simulink model "Droop_Ctrl"  (R2022b)
settings: Solver=ode113  StartTime=0.0  StopTime=1.5  RelTol=1e-3  EnableMultiTasking=on
libraries: spsSeriesRLCBranchLib x12, powerlib_extras x11, spsThreePhaseVIMeasurementLib x8, spsThreePhaseBreakerLib x7, spsThreePhaseSeriesRLCLoadLib x4, spsabctodq0Lib x4, spsDCVoltageSourceLib x2, spsThreePhaseSeriesRLCBranchLib x2, spsUniversalBridgeLib x2, spsdq0toabcLib x1, spspowerguiLib x1
settings Model: SimulationMode=accelerator  Creator=Administrator  LastModifiedBy=Rov
settings SolverCC: AlgebraicLoopSolver=TrustRegion
settings DataIOCC: LimitDataPoints=on  SaveFormat=Array  ReturnWorkspaceOutputs=off
settings OptimizationCC: ExpressionDepthLimit=2147483647  LifeSpan=inf
settings DebuggingCC: UnderspecifiedInitializationDetection=Classic  MergeDetectMultiDrivingBlocksExec=none  SolverPrmCheckMsg=warning  UnconnectedInputMsg=warning  UnconnectedOutputMsg=warning  UnconnectedLineMsg=warning  AllowSymbolicDim=off  StateNameClashWarn=warning  SFUnexpectedBacktrackingDiag=warning  SFNoUnconditionalDefaultTransitionDiag=warning  SFExecutionAtInitializationDiag=none  SFMachineParentedDataDiag=warning  ArithmeticOperatorsInVariantConditions=warning
settings HardwareCC: ProdBitPerPointer=32  ProdBitPerSizeT=32  ProdBitPerPtrDiffT=32  ProdLargestAtomicFloat=None  ProdIntDivRoundTo=Undefined  ProdEndianess=Unspecified  ProdWordSize=32  ProdHWDeviceType=32-bit Generic
settings ModelReferenceCC: EnableRefExpFcnMdlSchedulingChecks=on  PropagateSignalLabelsOutOfModel=off
settings SFSimCC: SimUseLocalCustomCode=off  CustomCodeUndefinedFunction=UseInterfaceOnly
settings RTWCC: RTWUseLocalCustomCode=off
settings CodeAppCC: StateflowObjectComments=on
settings GRTTargetCC: TargetLangStandard=C89/C90 (ANSI)
settings ConfigComp: CovMetricSettings=dw  CovSaveCumulativeToWorkspaceVar=on  CovSaveSingleToWorkspaceVar=on  CovExternalEMLEnable=off
settings SimscapeCC: SimscapeNormalizeSystem=off

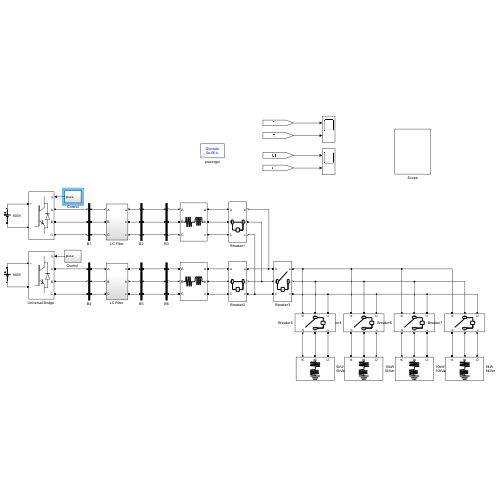
[thumbnail: Simulink's stored preview of the top-level diagram]
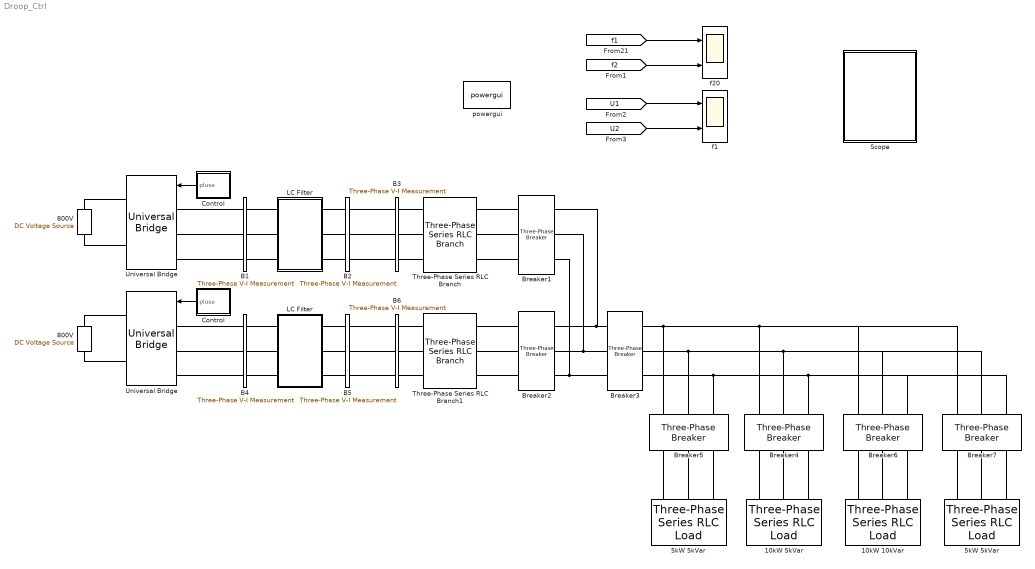
== system Droop_Ctrl ==
  10kW 10kVar : spsThreePhaseSeriesRLCLoadLib/Three-Phase Series RLC Load  LConnTagsString=A|B|C  Configuration=Y (grounded)  NominalVoltage=380  Vabc=[1e3 1e3 1e3]  Vabcp=[1e3 1e3 1e3]  NominalFrequency=50  UnbalancedPower=off  ActivePower=10e3  InductivePower=10e3  CapacitivePower=0  Pabc=[10e3 9e3 11e3]  QLabc=[100 90 110]  QCabc=[100 90 110]  Pabcp=[10e3 9e3 11e3]  QLabcp=[100 90 110]  QCabcp=[100 90 110]  Measurements=None  LoadType=constant Z
  10kW 5kVar : spsThreePhaseSeriesRLCLoadLib/Three-Phase Series RLC Load  LConnTagsString=A|B|C  Configuration=Y (grounded)  NominalVoltage=380  Vabc=[1e3 1e3 1e3]  Vabcp=[1e3 1e3 1e3]  NominalFrequency=50  UnbalancedPower=off  ActivePower=10e3  InductivePower=5e3  CapacitivePower=0  Pabc=[10e3 9e3 11e3]  QLabc=[100 90 110]  QCabc=[100 90 110]  Pabcp=[10e3 9e3 11e3]  QLabcp=[100 90 110]  QCabcp=[100 90 110]  Measurements=None  LoadType=constant Z
  5kW 5kVar : spsThreePhaseSeriesRLCLoadLib/Three-Phase Series RLC Load  LConnTagsString=A|B|C  Configuration=Y (grounded)  NominalVoltage=380  Vabc=[1e3 1e3 1e3]  Vabcp=[1e3 1e3 1e3]  NominalFrequency=50  UnbalancedPower=off  ActivePower=5e3  InductivePower=5e3  CapacitivePower=0  Pabc=[10e3 9e3 11e3]  QLabc=[100 90 110]  QCabc=[100 90 110]  Pabcp=[10e3 9e3 11e3]  QLabcp=[100 90 110]  QCabcp=[100 90 110]  Measurements=None  LoadType=constant Z
  "5kW 5kVar " : spsThreePhaseSeriesRLCLoadLib/Three-Phase Series RLC Load  LConnTagsString=A|B|C  Configuration=Y (grounded)  NominalVoltage=380  Vabc=[1e3 1e3 1e3]  Vabcp=[1e3 1e3 1e3]  NominalFrequency=50  UnbalancedPower=off  ActivePower=5e3  InductivePower=5e3  CapacitivePower=0  Pabc=[10e3 9e3 11e3]  QLabc=[100 90 110]  QCabc=[100 90 110]  Pabcp=[10e3 9e3 11e3]  QLabcp=[100 90 110]  QCabcp=[100 90 110]  Measurements=None  LoadType=constant Z
  800V : spsDCVoltageSourceLib/DC Voltage Source  Amplitude=800  Measurements=None
  "800V " : spsDCVoltageSourceLib/DC Voltage Source  Amplitude=800  Measurements=None
  B1 : spsThreePhaseVIMeasurementLib/Three-Phase V-I Measurement  VoltageMeasurement=phase-to-ground  SetLabelV=on  LabelV=Vabc_B1  Vpu=off  VpuLL=off  CurrentMeasurement=yes  SetLabelI=on  LabelI=Iabc_B1  Ipu=off  Pbase=100e6  Vbase=500e3  OutputType=Complex  PhasorSimulation=off  PSBequivalent=0
  B2 : spsThreePhaseVIMeasurementLib/Three-Phase V-I Measurement  VoltageMeasurement=phase-to-ground  SetLabelV=on  LabelV=Vabc_B2  Vpu=off  VpuLL=off  CurrentMeasurement=yes  SetLabelI=on  LabelI=Iabc_B2  Ipu=off  Pbase=100e6  Vbase=500e3  OutputType=Complex  PhasorSimulation=off  PSBequivalent=0
  B3 : spsThreePhaseVIMeasurementLib/Three-Phase V-I Measurement  VoltageMeasurement=phase-to-ground  SetLabelV=on  LabelV=Vabc_B3  Vpu=off  VpuLL=off  CurrentMeasurement=yes  SetLabelI=on  LabelI=Iabc_B3  Ipu=off  Pbase=100e6  Vbase=500e3  OutputType=Complex  PhasorSimulation=off  PSBequivalent=0
  B4 : spsThreePhaseVIMeasurementLib/Three-Phase V-I Measurement  VoltageMeasurement=phase-to-ground  SetLabelV=on  LabelV=Vabc_B4  Vpu=off  VpuLL=off  CurrentMeasurement=yes  SetLabelI=on  LabelI=Iabc_B4  Ipu=off  Pbase=100e6  Vbase=500e3  OutputType=Complex  PhasorSimulation=off  PSBequivalent=0
  B5 : spsThreePhaseVIMeasurementLib/Three-Phase V-I Measurement  VoltageMeasurement=phase-to-ground  SetLabelV=on  LabelV=Vabc_B5  Vpu=off  VpuLL=off  CurrentMeasurement=yes  SetLabelI=on  LabelI=Iabc_B5  Ipu=off  Pbase=100e6  Vbase=500e3  OutputType=Complex  PhasorSimulation=off  PSBequivalent=0
  B6 : spsThreePhaseVIMeasurementLib/Three-Phase V-I Measurement  VoltageMeasurement=phase-to-ground  SetLabelV=on  LabelV=Vabc_B6  Vpu=off  VpuLL=off  CurrentMeasurement=yes  SetLabelI=on  LabelI=Iabc_B6  Ipu=off  Pbase=100e6  Vbase=500e3  OutputType=Complex  PhasorSimulation=off  PSBequivalent=0
  Breaker1 : spsThreePhaseBreakerLib/Three-Phase Breaker  InitialState=closed  SwitchA=on  SwitchB=on  SwitchC=on  SwitchTimes=[10 10.4]  External=off  BreakerResistance=0.001  SnubberResistance=1e6  SnubberCapacitance=inf  Measurements=None
  Breaker2 : spsThreePhaseBreakerLib/Three-Phase Breaker  InitialState=closed  SwitchA=on  SwitchB=on  SwitchC=on  SwitchTimes=[10 10.4]  External=off  BreakerResistance=0.001  SnubberResistance=1e6  SnubberCapacitance=inf  Measurements=None
  Breaker3 : spsThreePhaseBreakerLib/Three-Phase Breaker  InitialState=open  SwitchA=on  SwitchB=on  SwitchC=on  SwitchTimes=[0.2 10]  External=off  BreakerResistance=0.001  SnubberResistance=1e6  SnubberCapacitance=inf  Measurements=None
  Breaker4 : spsThreePhaseBreakerLib/Three-Phase Breaker  InitialState=open  SwitchA=on  SwitchB=on  SwitchC=on  SwitchTimes=[0.4 0.6]  External=off  BreakerResistance=0.001  SnubberResistance=1e6  SnubberCapacitance=inf  Measurements=None
  Breaker5 : spsThreePhaseBreakerLib/Three-Phase Breaker  InitialState=open  SwitchA=on  SwitchB=on  SwitchC=on  SwitchTimes=[0.2 0.4]  External=off  BreakerResistance=0.001  SnubberResistance=1e6  SnubberCapacitance=inf  Measurements=None
  Breaker6 : spsThreePhaseBreakerLib/Three-Phase Breaker  InitialState=open  SwitchA=on  SwitchB=on  SwitchC=on  SwitchTimes=[0.6 0.8]  External=off  BreakerResistance=0.001  SnubberResistance=1e6  SnubberCapacitance=inf  Measurements=None
  Breaker7 : spsThreePhaseBreakerLib/Three-Phase Breaker  InitialState=open  SwitchA=on  SwitchB=on  SwitchC=on  SwitchTimes=[0.8 1]  External=off  BreakerResistance=0.001  SnubberResistance=1e6  SnubberCapacitance=inf  Measurements=None
  Control : Subsystem
  "Control " : Subsystem
  LC Filter : Subsystem
  "LC Filter " : Subsystem
  Scope : Subsystem
  Three-Phase Series RLC Branch : spsThreePhaseSeriesRLCBranchLib/Three-Phase Series RLC Branch  LConnTagsString=A|B|C  RConnTagsString=A|B|C  BranchType=RL  Resistance=0.642/5  Inductance=0.37e-3  Capacitance=1e-6  Measurements=None
  Three-Phase Series RLC Branch1 : spsThreePhaseSeriesRLCBranchLib/Three-Phase Series RLC Branch  LConnTagsString=A|B|C  RConnTagsString=A|B|C  BranchType=RL  Resistance=0.642/5  Inductance=0.37e-3  Capacitance=1e-6  Measurements=None
  Universal Bridge : spsUniversalBridgeLib/Universal Bridge  Arms=3  SnubberResistance=1e5  SnubberCapacitance=inf  Device=IGBT / Diodes  Ron=1e-3  Lon=0  ForwardVoltages="[  0  0  ]"  ForwardVoltage=0  GTOparameters=[ 10e-6 , 20e-6 ]  IGBTparameters=[ 1e-6 , 2e-6 ]  Measurements=None  Measurements_2=None  converterType=Rectifier
  "Universal Bridge " : spsUniversalBridgeLib/Universal Bridge  Arms=3  SnubberResistance=1e5  SnubberCapacitance=inf  Device=IGBT / Diodes  Ron=1e-3  Lon=0  ForwardVoltages="[  0  0  ]"  ForwardVoltage=0  GTOparameters=[ 10e-6 , 20e-6 ]  IGBTparameters=[ 1e-6 , 2e-6 ]  Measurements=None  Measurements_2=None  converterType=Rectifier
  f1 : Scope  NumInputPorts=2
  f20 : Scope  NumInputPorts=2
  powergui : spspowerguiLib/powergui  Priority=1  SimulationMode=Discrete  SampleTime=5e-6  frequency=60  Iterations=50  frequencyindice=0  Pbase=100e6  ErrMax=1e-4  UnitsV=kV  UnitsW=MW  buscounter=0  FunctionMessages=off  echomessages=off  EnableUseOfTLC=off  CurrentSourceSwitches=off  DisableSnubberDevices=off  DisableRonSwitches=off  DisableVfSwitches=off  DisplayEquations=off  AutomaticDiscreteSolvers=off  SolverType=Tustin  Interpol=off  ExternalGateDelay=off  methode=off  Ts=100  x0status=blocks  SPID=off  SwTol=0  HookPort=off  NonlinearTolerance=1e-4  nMaxIteration=100  ContinueOnMaxIteration=off  RestoreLinks=warning  ResistiveCurrentMeasurement=off  Frange=[0:2:500]  Ylog=off  Xlog=on  ShowGrid=off  save=off  variable=ZData  structure=0  ZoomFFT=off  StartTime=0.0  cycles=1  DisplayStyle=1  fundamental=60  FreqAxis=off  MaxFrequency=1000  frequencyindicesteady=1  RmsSteady=1  display=off
  wires:
  Control/1(pluse) -> Universal Bridge/1
  "Control "/1(pluse) -> "Universal Bridge "/1
  [f1] -> f20/1
  [f2] -> f20/2
  [U1] -> f1/1
  [U2] -> f1/2
  connections:
  B2/RConn3 -- B3/LConn3
  B2/RConn2 -- B3/LConn2
  B2/RConn1 -- B3/LConn1
  800V/LConn1 -- Universal Bridge/RConn2
  800V/RConn1 -- Universal Bridge/RConn1
  Universal Bridge/LConn1 -- B1/LConn1
  Universal Bridge/LConn2 -- B1/LConn2
  Universal Bridge/LConn3 -- B1/LConn3
  Three-Phase Series RLC Branch/LConn3 -- B3/RConn3
  Three-Phase Series RLC Branch/LConn2 -- B3/RConn2
  Three-Phase Series RLC Branch/LConn1 -- B3/RConn1
  B1/RConn1 -- LC Filter/LConn1
  B2/LConn1 -- LC Filter/RConn1
  B1/RConn2 -- LC Filter/LConn2
  B2/LConn2 -- LC Filter/RConn2
  B1/RConn3 -- LC Filter/LConn3
  B2/LConn3 -- LC Filter/RConn3
  B5/RConn3 -- B6/LConn3
  B5/RConn2 -- B6/LConn2
  B5/RConn1 -- B6/LConn1
  B5/LConn3 -- "LC Filter "/RConn3
  Three-Phase Series RLC Branch1/LConn1 -- B6/RConn1
  Three-Phase Series RLC Branch1/LConn3 -- B6/RConn3
  "Universal Bridge "/LConn1 -- B4/LConn1
  "Universal Bridge "/LConn3 -- B4/LConn3
  B4/RConn1 -- "LC Filter "/LConn1
  "800V "/LConn1 -- "Universal Bridge "/RConn2
  B5/LConn2 -- "LC Filter "/RConn2
  "Universal Bridge "/LConn2 -- B4/LConn2
  Three-Phase Series RLC Branch1/LConn2 -- B6/RConn2
  "800V "/RConn1 -- "Universal Bridge "/RConn1
  B5/LConn1 -- "LC Filter "/RConn1
  B4/RConn2 -- "LC Filter "/LConn2
  B4/RConn3 -- "LC Filter "/LConn3
  Breaker2/RConn1 -- Breaker1/RConn1 -- Breaker3/LConn1
  Breaker1/RConn2 -- Breaker3/LConn2 -- Breaker2/RConn2
  Breaker1/RConn3 -- Breaker3/LConn3 -- Breaker2/RConn3
  Breaker1/LConn1 -- Three-Phase Series RLC Branch/RConn1
  Breaker1/LConn2 -- Three-Phase Series RLC Branch/RConn2
  Breaker1/LConn3 -- Three-Phase Series RLC Branch/RConn3
  Breaker2/LConn1 -- Three-Phase Series RLC Branch1/RConn1
  Breaker2/LConn2 -- Three-Phase Series RLC Branch1/RConn2
  Breaker2/LConn3 -- Three-Phase Series RLC Branch1/RConn3
  10kW 5kVar/LConn1 -- Breaker4/RConn1
  10kW 5kVar/LConn2 -- Breaker4/RConn2
  10kW 5kVar/LConn3 -- Breaker4/RConn3
  5kW 5kVar/LConn2 -- Breaker5/RConn2
  5kW 5kVar/LConn3 -- Breaker5/RConn3
  5kW 5kVar/LConn1 -- Breaker5/RConn1
  Breaker3/RConn1 -- Breaker7/LConn1 -- Breaker6/LConn1 -- Breaker4/LConn1 -- Breaker5/LConn1
  Breaker3/RConn2 -- Breaker7/LConn2 -- Breaker6/LConn2 -- Breaker4/LConn2 -- Breaker5/LConn2
  Breaker3/RConn3 -- Breaker5/LConn3 -- Breaker4/LConn3 -- Breaker6/LConn3 -- Breaker7/LConn3
  10kW 10kVar/LConn3 -- Breaker6/RConn3
  10kW 10kVar/LConn2 -- Breaker6/RConn2
  10kW 10kVar/LConn1 -- Breaker6/RConn1
  "5kW 5kVar "/LConn1 -- Breaker7/RConn1
  "5kW 5kVar "/LConn2 -- Breaker7/RConn2
  "5kW 5kVar "/LConn3 -- Breaker7/RConn3

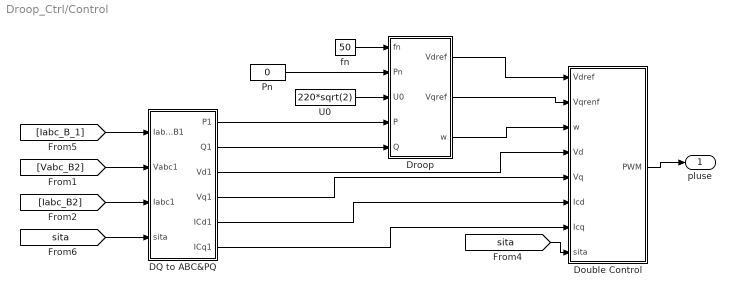
== system Droop_Ctrl/Control ==
  DQ to ABC&PQ : Subsystem
  Double Control : Subsystem
  Droop : Subsystem
  Pn : Constant  Value=0
  U0 : Constant  Value=220*sqrt(2)
  fn : Constant  Value=50
  pluse : Outport  VectorParamsAs1DForOutWhenUnconnected=off
  wires:
  Droop/3(w) -> Double Control/3(w)
  Double Control/1(PWM) -> pluse/1
  Droop/2(Vqref) -> Double Control/2(Vqrenf)
  Droop/1(Vdref) -> Double Control/1(Vdref)
  Pn/1 -> Droop/2(Pn)
  U0/1 -> Droop/3(U0)
  fn/1 -> Droop/1(fn)
  [sita] -> Double Control/8(sita)
  [sita] -> DQ to ABC&PQ/4(sita)
  [Vabc_B2] -> DQ to ABC&PQ/2(Vabc1)
  [Iabc_B2] -> DQ to ABC&PQ/3(Iabc1)
  [Iabc_B_1] -> DQ to ABC&PQ/1(Iabc_B1)
  DQ to ABC&PQ/6(ICq1) -> Double Control/7(Icq)
  DQ to ABC&PQ/5(ICd1) -> Double Control/6(Icd)
  DQ to ABC&PQ/4(Vq1) -> Double Control/5(Vq)
  DQ to ABC&PQ/3(Vd1) -> Double Control/4(Vd)
  DQ to ABC&PQ/2(Q1) -> Droop/5(Q)
  DQ to ABC&PQ/1(P1) -> Droop/4(P)

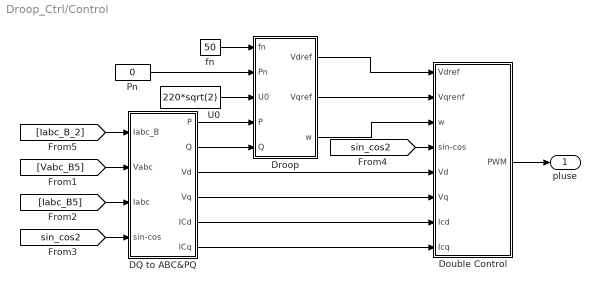
== system Droop_Ctrl/Control  ==
  DQ to ABC&PQ : Subsystem
  Double Control : Subsystem
  Droop : Subsystem
  Pn : Constant  Value=0
  U0 : Constant  Value=220*sqrt(2)
  fn : Constant  Value=50
  pluse : Outport  VectorParamsAs1DForOutWhenUnconnected=off
  wires:
  DQ to ABC&PQ/5(ICd) -> Double Control/7(Icd)
  Droop/3(w) -> Double Control/3(w)
  Double Control/1(PWM) -> pluse/1
  Droop/2(Vqref) -> Double Control/2(Vqrenf)
  Droop/1(Vdref) -> Double Control/1(Vdref)
  DQ to ABC&PQ/3(Vd) -> Double Control/5(Vd)
  DQ to ABC&PQ/6(ICq) -> Double Control/8(Icq)
  Pn/1 -> Droop/2(Pn)
  U0/1 -> Droop/3(U0)
  [Vabc_B5] -> DQ to ABC&PQ/2(Vabc)
  DQ to ABC&PQ/4(Vq) -> Double Control/6(Vq)
  DQ to ABC&PQ/1(P) -> Droop/4(P)
  [Iabc_B_2] -> DQ to ABC&PQ/1(Iabc_B)
  fn/1 -> Droop/1(fn)
  DQ to ABC&PQ/2(Q) -> Droop/5(Q)
  [Iabc_B5] -> DQ to ABC&PQ/3(Iabc)
  [sin_cos2] -> DQ to ABC&PQ/4(sin-cos)
  [sin_cos2] -> Double Control/4(sin-cos)

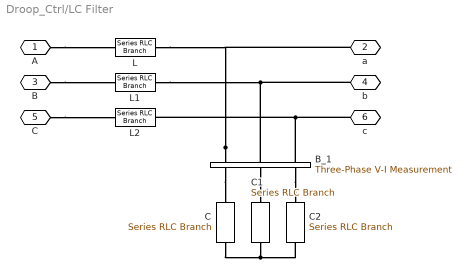
== system Droop_Ctrl/LC Filter ==
  " B_1" : spsThreePhaseVIMeasurementLib/Three-Phase V-I Measurement  VoltageMeasurement=phase-to-ground  SetLabelV=on  LabelV=Vabc_B_1  Vpu=off  VpuLL=off  CurrentMeasurement=yes  SetLabelI=on  LabelI=Iabc_B_1  Ipu=off  Pbase=100e6  Vbase=500e3  OutputType=Complex  PhasorSimulation=off  PSBequivalent=0
  C : spsSeriesRLCBranchLib/Series RLC Branch  LConnTagsString=__new0  RConnTagsString=__new0  BranchType=C  Resistance=0.01  Inductance=1e-3  SetiL0=off  InitialCurrent=0  Capacitance=1500e-6  Setx0=off  InitialVoltage=0  Measurements=None
  C1 : spsSeriesRLCBranchLib/Series RLC Branch  LConnTagsString=__new0  RConnTagsString=__new0  BranchType=C  Resistance=0.01  Inductance=1e-3  SetiL0=off  InitialCurrent=0  Capacitance=1500e-6  Setx0=off  InitialVoltage=0  Measurements=None
  C2 : spsSeriesRLCBranchLib/Series RLC Branch  LConnTagsString=__new0  RConnTagsString=__new0  BranchType=C  Resistance=0.01  Inductance=1e-3  SetiL0=off  InitialCurrent=0  Capacitance=1500e-6  Setx0=off  InitialVoltage=0  Measurements=None
  L : spsSeriesRLCBranchLib/Series RLC Branch  LConnTagsString=__new0  RConnTagsString=__new0  BranchType=L  Resistance=0.01  Inductance=2e-3  SetiL0=off  InitialCurrent=0  Capacitance=1e-6  Setx0=off  InitialVoltage=0  Measurements=None
  L1 : spsSeriesRLCBranchLib/Series RLC Branch  LConnTagsString=__new0  RConnTagsString=__new0  BranchType=L  Resistance=0.01  Inductance=2e-3  SetiL0=off  InitialCurrent=0  Capacitance=1e-6  Setx0=off  InitialVoltage=0  Measurements=None
  L2 : spsSeriesRLCBranchLib/Series RLC Branch  LConnTagsString=__new0  RConnTagsString=__new0  BranchType=L  Resistance=0.01  Inductance=2e-3  SetiL0=off  InitialCurrent=0  Capacitance=1e-6  Setx0=off  InitialVoltage=0  Measurements=None
  A : PMIOPort  Side=Left
  a : PMIOPort  Port=2  Side=Right
  B : PMIOPort  Port=3  Side=Left
  b : PMIOPort  Port=4  Side=Right
  "C " : PMIOPort  Port=5  Side=Left
  c : PMIOPort  Port=6  Side=Right
  connections:
  " B_1"/LConn1 -- a/RConn1 -- L/RConn1
  " B_1"/LConn3 -- c/RConn1 -- L2/RConn1
  A/RConn1 -- L/LConn1
  " B_1"/RConn2 -- C1/LConn1
  " B_1"/RConn3 -- C2/LConn1
  C1/RConn1 -- C/RConn1 -- C2/RConn1
  "C "/RConn1 -- L2/LConn1
  B/RConn1 -- L1/LConn1
  " B_1"/LConn2 -- b/RConn1 -- L1/RConn1
  " B_1"/RConn1 -- C/LConn1

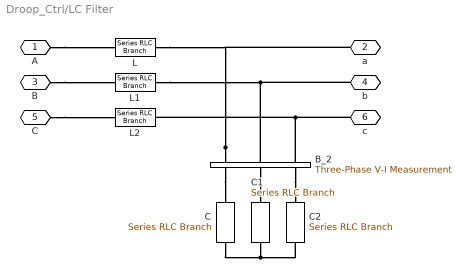
== system Droop_Ctrl/LC Filter  ==
  " B_2" : spsThreePhaseVIMeasurementLib/Three-Phase V-I Measurement  VoltageMeasurement=phase-to-ground  SetLabelV=on  LabelV=Vabc_B_2  Vpu=off  VpuLL=off  CurrentMeasurement=yes  SetLabelI=on  LabelI=Iabc_B_2  Ipu=off  Pbase=100e6  Vbase=500e3  OutputType=Complex  PhasorSimulation=off  PSBequivalent=0
  C : spsSeriesRLCBranchLib/Series RLC Branch  LConnTagsString=__new0  RConnTagsString=__new0  BranchType=C  Resistance=0.01  Inductance=1e-3  SetiL0=off  InitialCurrent=0  Capacitance=1500e-6  Setx0=off  InitialVoltage=0  Measurements=None
  C1 : spsSeriesRLCBranchLib/Series RLC Branch  LConnTagsString=__new0  RConnTagsString=__new0  BranchType=C  Resistance=0.01  Inductance=1e-3  SetiL0=off  InitialCurrent=0  Capacitance=1500e-6  Setx0=off  InitialVoltage=0  Measurements=None
  C2 : spsSeriesRLCBranchLib/Series RLC Branch  LConnTagsString=__new0  RConnTagsString=__new0  BranchType=C  Resistance=0.01  Inductance=1e-3  SetiL0=off  InitialCurrent=0  Capacitance=1500e-6  Setx0=off  InitialVoltage=0  Measurements=None
  L : spsSeriesRLCBranchLib/Series RLC Branch  LConnTagsString=__new0  RConnTagsString=__new0  BranchType=L  Resistance=0.01  Inductance=2e-3  SetiL0=off  InitialCurrent=0  Capacitance=1e-6  Setx0=off  InitialVoltage=0  Measurements=None
  L1 : spsSeriesRLCBranchLib/Series RLC Branch  LConnTagsString=__new0  RConnTagsString=__new0  BranchType=L  Resistance=0.01  Inductance=2e-3  SetiL0=off  InitialCurrent=0  Capacitance=1e-6  Setx0=off  InitialVoltage=0  Measurements=None
  L2 : spsSeriesRLCBranchLib/Series RLC Branch  LConnTagsString=__new0  RConnTagsString=__new0  BranchType=L  Resistance=0.01  Inductance=2e-3  SetiL0=off  InitialCurrent=0  Capacitance=1e-6  Setx0=off  InitialVoltage=0  Measurements=None
  A : PMIOPort  Side=Left
  a : PMIOPort  Port=2  Side=Right
  B : PMIOPort  Port=3  Side=Left
  b : PMIOPort  Port=4  Side=Right
  "C " : PMIOPort  Port=5  Side=Left
  c : PMIOPort  Port=6  Side=Right
  connections:
  " B_2"/LConn1 -- a/RConn1 -- L/RConn1
  " B_2"/LConn3 -- c/RConn1 -- L2/RConn1
  A/RConn1 -- L/LConn1
  " B_2"/RConn2 -- C1/LConn1
  " B_2"/RConn3 -- C2/LConn1
  C1/RConn1 -- C/RConn1 -- C2/RConn1
  "C "/RConn1 -- L2/LConn1
  B/RConn1 -- L1/LConn1
  " B_2"/LConn2 -- b/RConn1 -- L1/RConn1
  " B_2"/RConn1 -- C/LConn1

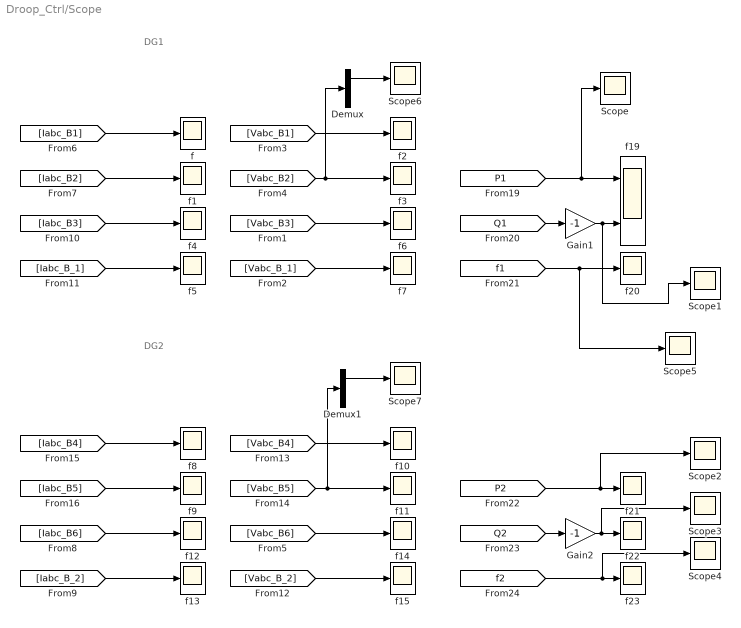
== system Droop_Ctrl/Scope ==
  note: DG1
  note: DG2
  Demux : Demux  Outputs=3
  Demux1 : Demux  Outputs=3
  Gain1 : Gain  Gain=-1
  Gain2 : Gain  Gain=-1
  Scope{,1..7} (8 alike) : Scope
  f{,1..15,20..23} (20 alike) : Scope
  f19 : Scope  NumInputPorts=2
  wires:
  [Vabc_B1] -> f2/1
  [Iabc_B3] -> f4/1
  [Vabc_B2] -> f3/1, Demux/1
  [Iabc_B1] -> f/1
  [Iabc_B2] -> f1/1
  [Iabc_B_1] -> f5/1
  [Vabc_B3] -> f6/1
  [Vabc_B_1] -> f7/1
  [Iabc_B4] -> f8/1
  [Vabc_B4] -> f10/1
  [Vabc_B6] -> f14/1
  [Iabc_B6] -> f12/1
  [Iabc_B5] -> f9/1
  [Iabc_B_2] -> f13/1
  [Vabc_B_2] -> f15/1
  [Q1] -> Gain1/1
  [P1] -> Scope/1, f19/1
  Gain1/1 -> Scope1/1, f19/2
  [f1] -> Scope5/1, f20/1
  [Q2] -> Gain2/1
  [P2] -> Scope2/1, f21/1
  Gain2/1 -> Scope3/1, f22/1
  [f2] -> Scope4/1, f23/1
  Demux/1 -> Scope6/1
  Demux1/1 -> Scope7/1
  [Vabc_B5] -> f11/1, Demux1/1

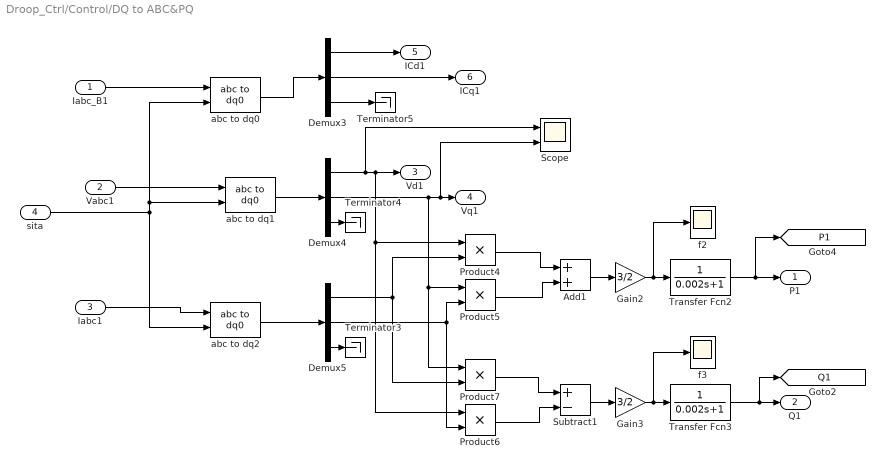
== system Droop_Ctrl/Control/DQ to ABC&PQ ==
  Iabc_B1 : Inport
  Vabc1 : Inport  Port=2
  Iabc1 : Inport  Port=3
  sita : Inport  Port=4
  Add1 : Sum
  Demux3 : Demux  Outputs=3
  Demux4 : Demux  Outputs=3
  Demux5 : Demux  Outputs=3
  Gain2 : Gain  Gain=3/2
  Gain3 : Gain  Gain=3/2
  Product{4..7} (4 alike) : Product  RndMeth=Zero
  Scope : Scope  NumInputPorts=2
  Subtract1 : Sum  Inputs=+-
  Terminator3 : Terminator
  Terminator4 : Terminator
  Terminator5 : Terminator
  Transfer Fcn2 : TransferFcn  Denominator=[0.002 1]
  Transfer Fcn3 : TransferFcn  Denominator=[0.002 1]
  abc to dq0 : spsabctodq0Lib/abc to dq0  Alignment=90 degrees behind phase A axis
  abc to dq1 : spsabctodq0Lib/abc to dq0  Alignment=90 degrees behind phase A axis
  abc to dq2 : spsabctodq0Lib/abc to dq0  Alignment=90 degrees behind phase A axis
  f2 : Scope
  f3 : Scope
  P1 : Outport  VectorParamsAs1DForOutWhenUnconnected=off
  Q1 : Outport  Port=2  VectorParamsAs1DForOutWhenUnconnected=off
  Vd1 : Outport  Port=3  VectorParamsAs1DForOutWhenUnconnected=off
  Vq1 : Outport  Port=4  VectorParamsAs1DForOutWhenUnconnected=off
  ICd1 : Outport  Port=5  VectorParamsAs1DForOutWhenUnconnected=off
  ICq1 : Outport  Port=6  VectorParamsAs1DForOutWhenUnconnected=off
  tag scope: P1=global, Q1=global
  wires:
  Demux3/3 -> Terminator5/1
  Demux5/1 -> Product7/2, Product4/2
  Add1/1 -> Gain2/1
  Gain3/1 -> f3/1, Transfer Fcn3/1
  Demux3/2 -> ICq1/1
  Product4/1 -> Add1/1
  Demux4/2 -> Scope/2, Vq1/1, Product7/1, Product5/1
  Vabc1/1 -> abc to dq1/1
  Product5/1 -> Add1/2
  abc to dq2/1 -> Demux5/1
  Demux4/1 -> Scope/1, Vd1/1, Product6/1, Product4/1
  Demux5/3 -> Terminator3/1
  Demux3/1 -> ICd1/1
  Demux4/3 -> Terminator4/1
  Gain2/1 -> f2/1, Transfer Fcn2/1
  Iabc_B1/1 -> abc to dq0/1
  Transfer Fcn2/1 -> [P1], P1/1
  Transfer Fcn3/1 -> [Q1], Q1/1
  Product7/1 -> Subtract1/1
  Product6/1 -> Subtract1/2
  abc to dq0/1 -> Demux3/1
  Demux5/2 -> Product6/2, Product5/2
  Subtract1/1 -> Gain3/1
  abc to dq1/1 -> Demux4/1
  sita/1 -> abc to dq2/2, abc to dq1/2, abc to dq0/2
  Iabc1/1 -> abc to dq2/1

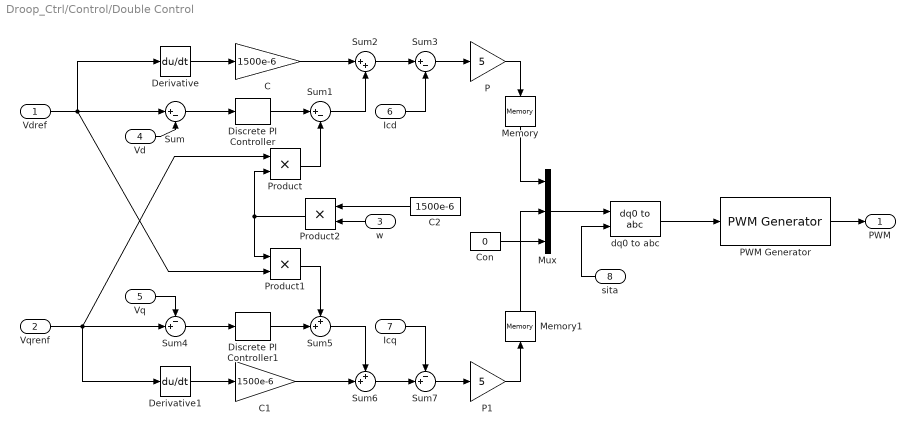
== system Droop_Ctrl/Control/Double Control ==
  Vdref : Inport
  Vqrenf : Inport  Port=2
  w : Inport  Port=3
  Vd : Inport  Port=4
  Vq : Inport  Port=5
  Icd : Inport  Port=6
  Icq : Inport  Port=7
  sita : Inport  Port=8
  C : Gain  Gain=1500e-6
  C1 : Gain  Gain=1500e-6
  C2 : Constant  Value=1500e-6
  Con : Constant  Value=0
  Derivative : Derivative
  Derivative1 : Derivative
  Discrete PI Controller : powerlib_extras/Discrete  Control Blocks/Discrete PI Controller  Kp=5  Ki=10  Par_Limits=[1e6 -1e6]  Init=0  Ts=50e-6
  Discrete PI Controller1 : powerlib_extras/Discrete  Control Blocks/Discrete PI Controller  Kp=5  Ki=10  Par_Limits=[1e6 -1e6]  Init=0  Ts=50e-6
  Memory : Memory
  Memory1 : Memory
  Mux : Mux  Inputs=3
  P : Gain  Gain=5
  P1 : Gain  Gain=5
  PWM Generator : powerlib_extras/Control  Blocks/PWM Generator  GeneratorMode="3-arm  bridge (6 pulses)"  Fc=1e+4  Internal=off  mIndex=0.4  Freq=60  Phase=0
  Product : Product  RndMeth=Zero
  Product1 : Product  RndMeth=Zero
  Product2 : Product  RndMeth=Zero
  Sum : Sum  Inputs=|+-
  Sum1 : Sum  Inputs=|+-
  Sum2 : Sum  Inputs=|++
  Sum3 : Sum  Inputs=|+-
  Sum4 : Sum  Inputs=-+|
  Sum5 : Sum  Inputs=++|
  Sum6 : Sum  Inputs=++|
  Sum7 : Sum  Inputs=-+|
  dq0 to abc : spsdq0toabcLib/dq0 to abc  Alignment=90 degrees behind phase A axis
  PWM : Outport  VectorParamsAs1DForOutWhenUnconnected=off
  wires:
  Discrete PI Controller/1 -> Sum1/1
  Con/1 -> Mux/3
  Vdref/1 -> Derivative/1, Sum/1, Product1/2
  Vd/1 -> Sum/2
  Icd/1 -> Sum3/2
  C/1 -> Sum2/1
  Sum2/1 -> Sum3/1
  Sum/1 -> Discrete PI Controller/1
  Sum1/1 -> Sum2/2
  Sum3/1 -> P/1
  Derivative/1 -> C/1
  Product/1 -> Sum1/2
  PWM Generator/1 -> PWM/1
  P/1 -> Memory/1
  Discrete PI Controller1/1 -> Sum5/2
  Sum4/1 -> Discrete PI Controller1/1
  Vq/1 -> Sum4/1
  Vqrenf/1 -> Sum4/2, Product/1, Derivative1/1
  Icq/1 -> Sum7/1
  P1/1 -> Memory1/1
  C1/1 -> Sum6/2
  Memory/1 -> Mux/1
  Sum7/1 -> P1/1
  Sum6/1 -> Sum7/2
  w/1 -> Product2/2
  Mux/1 -> dq0 to abc/1
  Derivative1/1 -> C1/1
  Memory1/1 -> Mux/2
  C2/1 -> Product2/1
  Product2/1 -> Product/2, Product1/1
  Product1/1 -> Sum5/1
  Sum5/1 -> Sum6/1
  sita/1 -> dq0 to abc/2
  dq0 to abc/1 -> PWM Generator/1

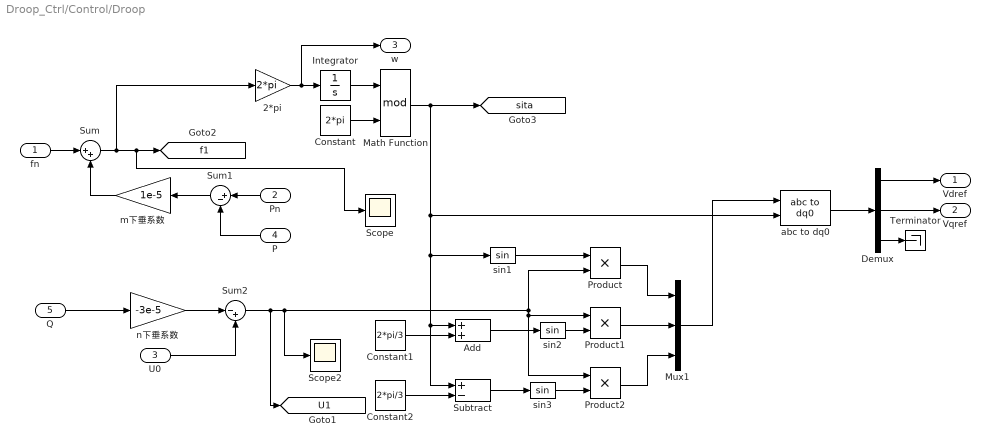
== system Droop_Ctrl/Control/Droop ==
  fn : Inport
  Pn : Inport  Port=2
  U0 : Inport  Port=3
  P : Inport  Port=4
  Q : Inport  Port=5
  2*pi : Gain  Gain=2*pi
  Add : Sum
  Constant : Constant  Value=2*pi
  Constant1 : Constant  Value=2*pi/3
  Constant2 : Constant  Value=2*pi/3
  Demux : Demux  Outputs=3
  Integrator : Integrator
  Math Function : Math  Operator=mod  SignedPower=on
  Mux1 : Mux  Inputs=3
  Product : Product  RndMeth=Zero
  Product1 : Product  RndMeth=Zero
  Product2 : Product  RndMeth=Zero
  Scope : Scope
  Scope2 : Scope
  Subtract : Sum  Inputs=+-
  Sum : Sum  Inputs=|++
  Sum1 : Sum  Inputs=|+-
  Sum2 : Sum  Inputs=|-+
  Terminator : Terminator
  abc to dq0 : spsabctodq0Lib/abc to dq0  Alignment=90 degrees behind phase A axis
  m下垂系数 : Gain  Gain=1e-5
  n下垂系数 : Gain  Gain=-3e-5
  sin1 : Trigonometry
  sin2 : Trigonometry
  sin3 : Trigonometry
  Vdref : Outport  VectorParamsAs1DForOutWhenUnconnected=off
  Vqref : Outport  Port=2  VectorParamsAs1DForOutWhenUnconnected=off
  w : Outport  Port=3  VectorParamsAs1DForOutWhenUnconnected=off
  tag scope: U1=global, f1=global, sita=global
  wires:
  Sum2/1 -> [U1], Scope2/1, Product2/1, Product1/1, Product/2
  Add/1 -> sin2/1
  Demux/1 -> Vdref/1
  fn/1 -> Sum/1
  P/1 -> Sum1/2
  2*pi/1 -> w/1, Integrator/1
  Math Function/1 -> abc to dq0/2, Subtract/1, Add/1, sin1/1, [sita]
  Constant2/1 -> Subtract/2
  Mux1/1 -> abc to dq0/1
  Sum/1 -> Scope/1, [f1], 2*pi/1
  m下垂系数/1 -> Sum/2
  Integrator/1 -> Math Function/1
  Sum1/1 -> m下垂系数/1
  Demux/3 -> Terminator/1
  Constant/1 -> Math Function/2
  Product2/1 -> Mux1/3
  n下垂系数/1 -> Sum2/1
  U0/1 -> Sum2/2
  Subtract/1 -> sin3/1
  Q/1 -> n下垂系数/1
  Demux/2 -> Vqref/1
  Product1/1 -> Mux1/2
  Constant1/1 -> Add/2
  Product/1 -> Mux1/1
  sin1/1 -> Product/1
  Pn/1 -> Sum1/1
  sin2/1 -> Product1/2
  sin3/1 -> Product2/2
  abc to dq0/1 -> Demux/1

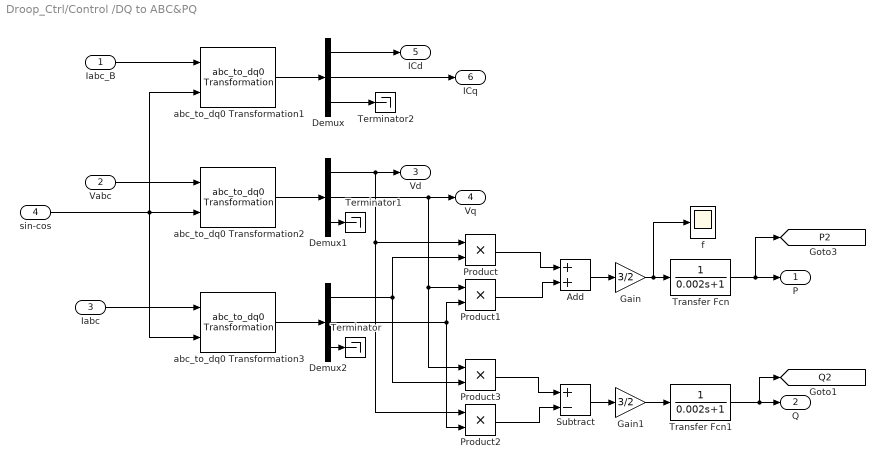
== system Droop_Ctrl/Control /DQ to ABC&PQ ==
  Iabc_B : Inport
  Vabc : Inport  Port=2
  Iabc : Inport  Port=3
  sin-cos : Inport  Port=4
  Add : Sum
  Demux : Demux  Outputs=3
  Demux1 : Demux  Outputs=3
  Demux2 : Demux  Outputs=3
  Gain : Gain  Gain=3/2
  Gain1 : Gain  Gain=3/2
  Product{,1..3} (4 alike) : Product  RndMeth=Zero
  Subtract : Sum  Inputs=+-
  Terminator : Terminator
  Terminator1 : Terminator
  Terminator2 : Terminator
  Transfer Fcn : TransferFcn  Denominator=[0.002 1]
  Transfer Fcn1 : TransferFcn  Denominator=[0.002 1]
  abc_to_dq0 Transformation1 : powerlib_extras/Measurements/abc_to_dq0 Transformation
  abc_to_dq0 Transformation2 : powerlib_extras/Measurements/abc_to_dq0 Transformation
  abc_to_dq0 Transformation3 : powerlib_extras/Measurements/abc_to_dq0 Transformation
  f : Scope
  P : Outport  VectorParamsAs1DForOutWhenUnconnected=off
  Q : Outport  Port=2  VectorParamsAs1DForOutWhenUnconnected=off
  Vd : Outport  Port=3  VectorParamsAs1DForOutWhenUnconnected=off
  Vq : Outport  Port=4  VectorParamsAs1DForOutWhenUnconnected=off
  ICd : Outport  Port=5  VectorParamsAs1DForOutWhenUnconnected=off
  ICq : Outport  Port=6  VectorParamsAs1DForOutWhenUnconnected=off
  tag scope: P2=global, Q2=global
  wires:
  abc_to_dq0 Transformation1/1 -> Demux/1
  abc_to_dq0 Transformation2/1 -> Demux1/1
  Demux/3 -> Terminator2/1
  abc_to_dq0 Transformation3/1 -> Demux2/1
  Demux1/3 -> Terminator1/1
  Demux2/3 -> Terminator/1
  sin-cos/1 -> abc_to_dq0 Transformation3/2, abc_to_dq0 Transformation1/2, abc_to_dq0 Transformation2/2
  Iabc_B/1 -> abc_to_dq0 Transformation1/1
  Iabc/1 -> abc_to_dq0 Transformation3/1
  Demux1/1 -> Vd/1, Product2/1, Product/1
  Demux/2 -> ICq/1
  Vabc/1 -> abc_to_dq0 Transformation2/1
  Demux1/2 -> Vq/1, Product3/1, Product1/1
  Demux/1 -> ICd/1
  Subtract/1 -> Gain1/1
  Add/1 -> Gain/1
  Demux2/2 -> Product2/2, Product1/2
  Demux2/1 -> Product3/2, Product/2
  Product3/1 -> Subtract/1
  Product1/1 -> Add/2
  Product/1 -> Add/1
  Gain1/1 -> Transfer Fcn1/1
  Product2/1 -> Subtract/2
  Gain/1 -> f/1, Transfer Fcn/1
  Transfer Fcn/1 -> [P2], P/1
  Transfer Fcn1/1 -> [Q2], Q/1

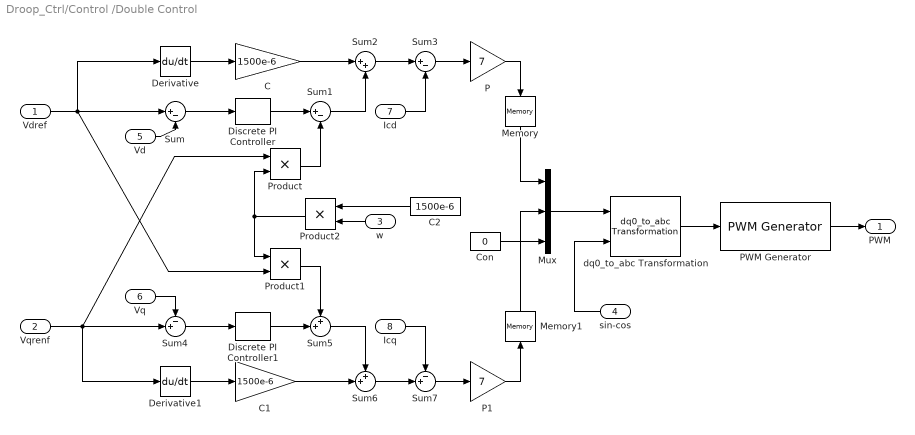
== system Droop_Ctrl/Control /Double Control ==
  Vdref : Inport
  Vqrenf : Inport  Port=2
  w : Inport  Port=3
  sin-cos : Inport  Port=4
  Vd : Inport  Port=5
  Vq : Inport  Port=6
  Icd : Inport  Port=7
  Icq : Inport  Port=8
  C : Gain  Gain=1500e-6
  C1 : Gain  Gain=1500e-6
  C2 : Constant  Value=1500e-6
  Con : Constant  Value=0
  Derivative : Derivative
  Derivative1 : Derivative
  Discrete PI Controller : powerlib_extras/Discrete  Control Blocks/Discrete PI Controller  Kp=5  Ki=10  Par_Limits=[1e6 -1e6]  Init=0  Ts=50e-6
  Discrete PI Controller1 : powerlib_extras/Discrete  Control Blocks/Discrete PI Controller  Kp=5  Ki=10  Par_Limits=[1e6 -1e6]  Init=0  Ts=50e-6
  Memory : Memory
  Memory1 : Memory
  Mux : Mux  Inputs=3
  P : Gain  Gain=7
  P1 : Gain  Gain=7
  PWM Generator : powerlib_extras/Control  Blocks/PWM Generator  GeneratorMode="3-arm  bridge (6 pulses)"  Fc=10000  Internal=off  mIndex=0.4  Freq=60  Phase=0
  Product : Product  RndMeth=Zero
  Product1 : Product  RndMeth=Zero
  Product2 : Product  RndMeth=Zero
  Sum : Sum  Inputs=|+-
  Sum1 : Sum  Inputs=|+-
  Sum2 : Sum  Inputs=|++
  Sum3 : Sum  Inputs=|+-
  Sum4 : Sum  Inputs=-+|
  Sum5 : Sum  Inputs=++|
  Sum6 : Sum  Inputs=++|
  Sum7 : Sum  Inputs=-+|
  dq0_to_abc Transformation : powerlib_extras/Measurements/dq0_to_abc Transformation
  PWM : Outport  VectorParamsAs1DForOutWhenUnconnected=off
  wires:
  sin-cos/1 -> dq0_to_abc Transformation/2
  Discrete PI Controller/1 -> Sum1/1
  Con/1 -> Mux/3
  Vdref/1 -> Derivative/1, Sum/1, Product1/2
  Vd/1 -> Sum/2
  Icd/1 -> Sum3/2
  C/1 -> Sum2/1
  Sum2/1 -> Sum3/1
  Sum/1 -> Discrete PI Controller/1
  Sum1/1 -> Sum2/2
  Sum3/1 -> P/1
  Derivative/1 -> C/1
  Product/1 -> Sum1/2
  PWM Generator/1 -> PWM/1
  P/1 -> Memory/1
  Discrete PI Controller1/1 -> Sum5/2
  Sum4/1 -> Discrete PI Controller1/1
  Vq/1 -> Sum4/1
  Vqrenf/1 -> Sum4/2, Product/1, Derivative1/1
  Icq/1 -> Sum7/1
  P1/1 -> Memory1/1
  C1/1 -> Sum6/2
  Memory/1 -> Mux/1
  Sum7/1 -> P1/1
  Sum6/1 -> Sum7/2
  w/1 -> Product2/2
  Mux/1 -> dq0_to_abc Transformation/1
  Derivative1/1 -> C1/1
  Memory1/1 -> Mux/2
  C2/1 -> Product2/1
  Product2/1 -> Product/2, Product1/1
  Product1/1 -> Sum5/1
  dq0_to_abc Transformation/1 -> PWM Generator/1
  Sum5/1 -> Sum6/1

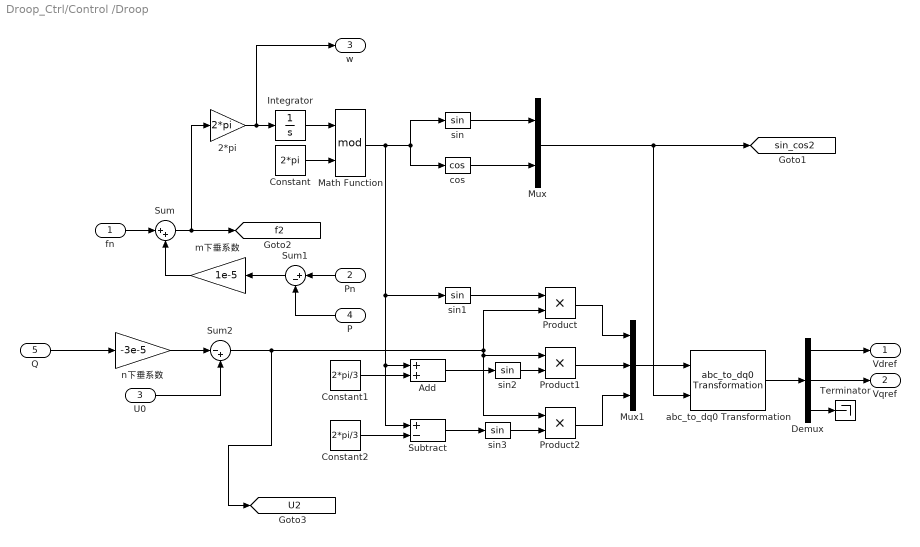
== system Droop_Ctrl/Control /Droop ==
  fn : Inport
  Pn : Inport  Port=2
  U0 : Inport  Port=3
  P : Inport  Port=4
  Q : Inport  Port=5
  2*pi : Gain  Gain=2*pi
  Add : Sum
  Constant : Constant  Value=2*pi
  Constant1 : Constant  Value=2*pi/3
  Constant2 : Constant  Value=2*pi/3
  Demux : Demux  Outputs=3
  Integrator : Integrator
  Math Function : Math  Operator=mod  SignedPower=on
  Mux : Mux  Inputs=2
  Mux1 : Mux  Inputs=3
  Product : Product  RndMeth=Zero
  Product1 : Product  RndMeth=Zero
  Product2 : Product  RndMeth=Zero
  Subtract : Sum  Inputs=+-
  Sum : Sum  Inputs=|++
  Sum1 : Sum  Inputs=|+-
  Sum2 : Sum  Inputs=|-+
  Terminator : Terminator
  abc_to_dq0 Transformation : powerlib_extras/Measurements/abc_to_dq0 Transformation
  cos : Trigonometry  Operator=cos
  m下垂系数 : Gain  Gain=1e-5
  n下垂系数 : Gain  Gain=-3e-5
  sin{,1..3} (4 alike) : Trigonometry
  Vdref : Outport  VectorParamsAs1DForOutWhenUnconnected=off
  Vqref : Outport  Port=2  VectorParamsAs1DForOutWhenUnconnected=off
  w : Outport  Port=3  VectorParamsAs1DForOutWhenUnconnected=off
  tag scope: U2=global, f2=global, sin_cos2=global
  wires:
  Sum2/1 -> [U2], Product2/1, Product1/1, Product/2
  Add/1 -> sin2/1
  Demux/1 -> Vdref/1
  fn/1 -> Sum/1
  cos/1 -> Mux/2
  P/1 -> Sum1/2
  2*pi/1 -> w/1, Integrator/1
  Math Function/1 -> Subtract/1, Add/1, sin1/1, cos/1, sin/1
  Constant2/1 -> Subtract/2
  Mux1/1 -> abc_to_dq0 Transformation/1
  Sum/1 -> [f2], 2*pi/1
  abc_to_dq0 Transformation/1 -> Demux/1
  m下垂系数/1 -> Sum/2
  Integrator/1 -> Math Function/1
  Mux/1 -> [sin_cos2], abc_to_dq0 Transformation/2
  Sum1/1 -> m下垂系数/1
  Demux/3 -> Terminator/1
  Constant/1 -> Math Function/2
  Product2/1 -> Mux1/3
  sin/1 -> Mux/1
  n下垂系数/1 -> Sum2/1
  U0/1 -> Sum2/2
  Subtract/1 -> sin3/1
  Q/1 -> n下垂系数/1
  Demux/2 -> Vqref/1
  Product1/1 -> Mux1/2
  Constant1/1 -> Add/2
  Product/1 -> Mux1/1
  sin1/1 -> Product/1
  Pn/1 -> Sum1/1
  sin2/1 -> Product1/2
  sin3/1 -> Product2/2
